simulink model "MBD3_problem2"  (R2020b)
settings: Solver=VariableStepAuto  StartTime=0.0  StopTime=150  RelTol=1e-3
settings Model: Creator=Lenovo  LastModifiedBy=Lenovo

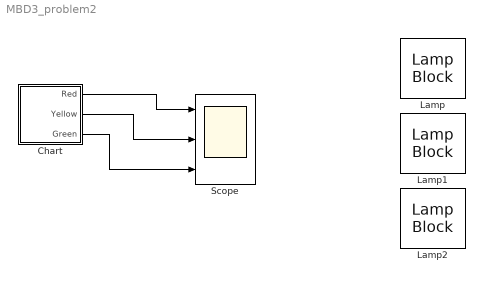
== system MBD3_problem2 ==
  Chart : Stateflow chart  TreatAsAtomicUnit=on
  Lamp : LampBlock
  Lamp1 : LampBlock
  Lamp2 : LampBlock
  Scope : Scope  NumInputPorts=3
  wires:
  Chart/1(Red) -> Scope/1
  Chart/2(Yellow) -> Scope/2
  Chart/3(Green) -> Scope/3

== stateflow chart MBD3_problem2/Chart ==
  state Stop
    entry:Red=1;
    Yellow=0;
    Green=0;
  state Ready_to_Start1
    during:Red=0;
    Yellow=1;
    Green=0;
  state Start
    during:Red=0;
    Yellow=0;
    Green=1;
  state Ready_to_Stop
    during:Red=0;
    Yellow=1;
    Green=0;
  (default) -> Stop
  Stop -> Ready_to_Start1 : after(10,sec)
  Ready_to_Start1 -> Start : after(60,sec)
  Start -> Ready_to_Stop : after(10,sec)
  Ready_to_Stop -> Stop : after(40,sec)
  data: Red output; Yellow output; Green output
